simulink model "CR_old"  (R2022a)
settings: Solver=FixedStepDiscrete  StartTime=0.0  StopTime=0.04  FixedStep=0.04  RelTol=1e-3
PreLoadFcn:
  | listing = dir;
  | if (contains([listing .name], 'AGR')) && (contains([listing .name], 'MAP'))
  |     addpath('./AGR', './MAP');
  |     addpath( genpath('./MAP') );
  | elseif (contains([listing .name], 'CR.slx'))
  |     addpath('../AGR', '../MAP');
  |     addpath( genpath('../MAP') );
  | else
  | 
  | end
  | 
  | load('BusStructureCR.mat');
InitFcn:
  | listing = dir;
  | if (contains([listing .name], 'AGR')) && (contains([listing .name], 'MAP'))
  |     addpath('./AGR', './MAP');
  |     addpath( genpath('./MAP') );
  | elseif (contains([listing .name], 'CR.slx'))
  |     addpath('../AGR', '../MAP');
  |     addpath( genpath('../MAP') );
  | else
  | 
  | end
  | 
  | load('BusStructureCR.mat');
StartFcn:
  | listing = dir;
  | if (contains([listing .name], 'AGR')) && (contains([listing .name], 'MAP'))
  |     addpath('./AGR', './MAP');
  |     addpath( genpath('./MAP') );
  | elseif (contains([listing .name], 'CR.slx'))
  |     addpath('../AGR', '../MAP');
  |     addpath( genpath('../MAP') );
  | else
  | 
  | end
  | 
  | load('BusStructureCR.mat');
undefined symbols (not defined in the file): CRDataTag, CRDataTagWrap, CRElevationValid, CRSelected, CRSelectedWraparound, CRTargetElevation, CRTargetLatitude, CRTargetLongitude, CRTargetLOSAvailable, CRTargetLOSAvailableValid, CRValid, deltaECEF, losECEF, nSearch, targetECEF, testLLH
settings Model: Creator=ASCL  LastModifiedBy=ASCL
settings SolverCC: AlgebraicLoopSolver=TrustRegion
settings DataIOCC: SaveOutput=off  SignalLogging=off  DSMLogging=off  SaveTime=off  ReturnWorkspaceOutputs=off
settings OptimizationCC: DefaultParameterBehavior=Inlined  UseDivisionForNetSlopeComputation=on  GainParamInheritBuiltInType=on  UseFloatMulNetSlope=on  InlineInvariantSignals=on  BufferReuse=off  ExpressionFolding=off  PassReuseOutputArgsAs=Individual arguments  ZeroExternalMemoryAtStartup=off  ZeroInternalMemoryAtStartup=off  NoFixptDivByZeroProtection=on  EfficientMapNaN2IntZero=off  LifeSpan=1  EfficientTunableParamExpr=on
settings DebuggingCC: ParameterTunabilityLossMsg=error  UnconnectedInputMsg=warning  UnconnectedOutputMsg=warning  UnconnectedLineMsg=warning  SFMachineParentedDataDiag=warning  ArithmeticOperatorsInVariantConditions=warning
settings HardwareCC: ProdBitPerPointer=32  ProdBitPerSizeT=32  ProdBitPerPtrDiffT=32  ProdLargestAtomicInteger=Long  ProdLargestAtomicFloat=Double  ProdEndianess=BigEndian  ProdWordSize=32  ProdLongLongMode=on  ProdHWDeviceType=Freescale->MPC83xx
settings ModelReferenceCC: ModelReferenceNumInstancesAllowed=Single
settings SFSimCC: SimUserLibraries=MAPd.lib WS2_32.lib  SimUseLocalCustomCode=off  MATLABDynamicMemAlloc=off  CustomCodeUndefinedFunction=UseInterfaceOnly
settings SFSimCC: SimCustomHeaderCode=|
  | #include "MAP.h"
  | #include "MAPDATA.h"
  | #include "DVOF.h"
  | #include "userDefined.h"
settings SFSimCC: SimUserSources=|
  | MAP.c
  | DVOF.c
  | userDefined.c
settings RTWCC: SystemTargetFile=ert.tlc  TemplateMakefile=ert_default_tmf  GenerateReport=on  RTWUseLocalCustomCode=off  RTWUseSimCustomCode=on  CustomLibrary=MAPd.lib WS2_32.lib  IncludeHyperlinkInReport=on  LaunchReport=on  GenerateTraceInfo=on  GenerateTraceReport=on  GenerateTraceReportSl=on  GenerateTraceReportSf=on  GenerateTraceReportEml=on  GenerateCodeMetricsReport=on
settings RTWCC: CustomHeaderCode=|
  | #include "MAP.h"
  | #include "MAPDATA.h"
  | #include "DVOF.h"
  | #include "userDefined.h"
settings RTWCC: CustomSource=|
  | MAP.c
  | DVOF.c
  | userDefined.c
settings CodeAppCC: ForceParamTrailComments=on  IgnoreCustomStorageClasses=off  OperatorAnnotations=on  SimulinkDataObjDesc=on  SFDataObjDesc=on  InsertBlockDesc=on
settings ERTTargetCC: TargetLangStandard=C99 (ISO)  UtilityFuncGeneration=Shared location  GenerateSampleERTMain=on  IncludeMdlTerminateFcn=off  CombineSignalStateStructs=on  SuppressErrorStatus=on  SupportAbsoluteTime=off  SupportComplex=off  InlinedParameterPlacement=NonHierarchical  ERTCustomFileTemplate=example_file_process.tlc  ERTFilePackagingFormat=CompactWithDataFile  EnableSignedLeftShifts=off  EnableSignedRightShifts=off

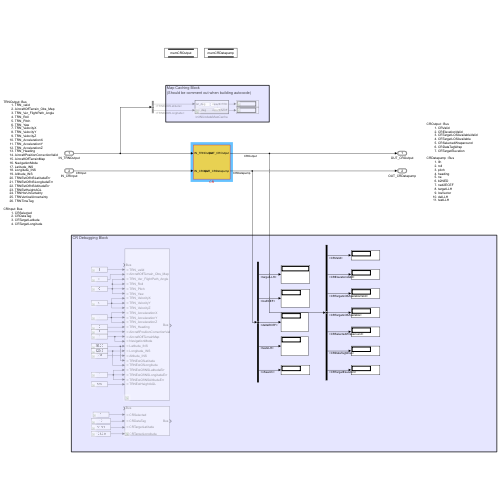
[thumbnail: Simulink's stored preview of the top-level diagram]
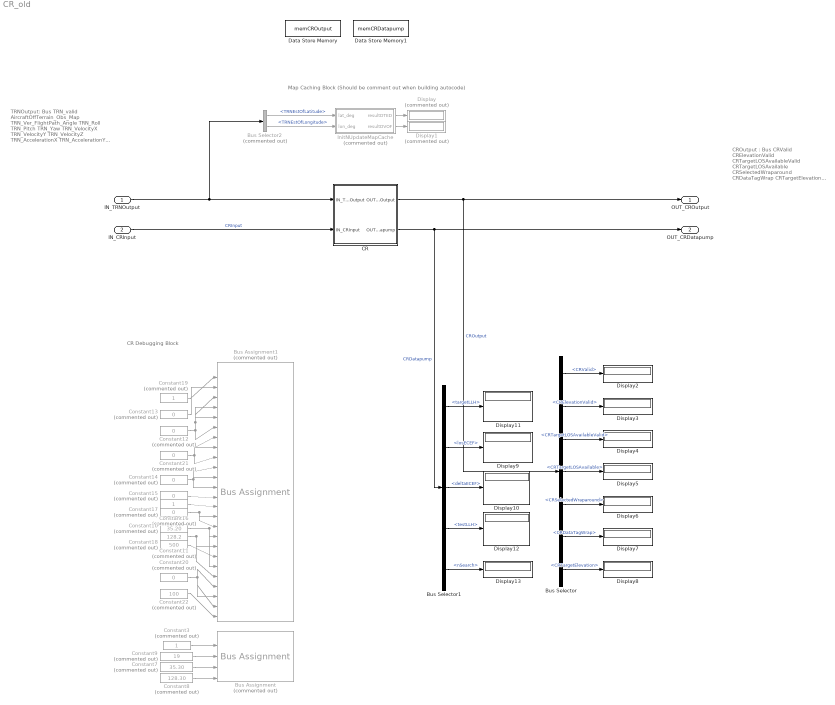
== system CR_old ==
  note: Map Caching Block
      | (Should be comment out when building autocode)
  note: TRNOutput: Bus
      | TRN_valid
      | AircraftOffTerrain_Obs_Map
      | TRN_Ver_FlightPath_Angle
      | TRN_Roll
      | TRN_Pitch
      | TRN_Yaw
      | TRN_VelocityX
      | TRN_VelocityY
      | TRN_VelocityZ
      | TRN_AccelerationX
      | TRN_AccelerationY
      | TRN_AccelerationZ
      | TRN_Heading
      | AircraftPositionCorrectionValid
      | AircraftOffTerrainMap
      | NavigationMode
      | Latitude_INS
      | Longitude_INS
      | Altitude_INS
      | TRNEstOfINSLatitudeErr
      | TRNEstOfINSLongitudeErr
      | TRNEstOfINSAltitudeErr
      | TRNEstHeightAGL
      | TRNHorUncertainty
      | TRNVerticalUncertainty
      | TRNTimeTag
      |
      | CRInput: Bus
      | CRSelected
      | CRDataTag
      | CRTargetLatitude
      | CRTargetLongitude
  note: CROutput : Bus
      | CRValid
      | CRElevationValid
      | CRTargetLOSAvailableValid
      | CRTargetLOSAvailable
      | CRSelectedWraparound
      | CRDataTagWrap
      | CRTargetElevation
      |
      | CRDatapump : Bus
      | llh
      | roll
      | pitch
      | heading
      | ne
      | b2NED
      | ned2ECEF
      | targetLLH
      | losVector
      | delLLH
      | testLLH
  note: CR Debugging Block
  IN_TRNOutput : Inport  OutDataTypeStr=Bus: TRNOutput  BusOutputAsStruct=on
  IN_CRInput : Inport  Port=2  OutDataTypeStr=Bus: CRInput  BusOutputAsStruct=on
  Bus Assignment : BusAssignment  Commented=on  AssignedSignals=CRSelected,CRDataTag,CRTargetLatitude,CRTargetLongitude
  Bus Assignment1 : BusAssignment  Commented=on  AssignedSignals=TRN_valid,AircraftOffTerrain_Obs_Map,TRN_Ver_FlightPath_Angle,TRN_Roll,TRN_Pitch,TRN_Yaw,TRN_VelocityX,TRN_VelocityY,TRN_VelocityZ,TRN_AccelerationX,TRN_AccelerationY,TRN_AccelerationZ,TRN_Heading,AircraftPositionCorrectionValid,AircraftOffTerrainMap,NavigationMode,Latitude_INS,Longitude_INS,Altitude_INS,TRNEstOfLatitude,TRNEstOfLongitude,TRNEstOfINSLatitudeErr,TRNEstOfINSLongitudeErr,TRNEstOfINSAltitudeErr,TRNEstHeightAGL
  Bus Selector : BusSelector  OutputSignals=CRValid,CRElevationValid,CRTargetLOSAvailableValid,CRTargetLOSAvailable,CRSelectedWraparound,CRDataTagWrap,CRTargetElevation
  Bus Selector1 : BusSelector  OutputSignals=targetLLH,losECEF,deltaECEF,testLLH,nSearch
  Bus Selector2 : BusSelector  Commented=on  OutputSignals=TRNEstOfLatitude,TRNEstOfLongitude
  CR : Subsystem
      mask init:
      | % latGPS = double(0);
      | % lonGPS = double(0);
      | % altGPS = double(0);
      | % velEGPS = double(0);
      | % velNGPS = double(0);
      | % velUGPS = double(0);
      | % notValidGPS = boolean(0);
      | % notAvaildINS = boolean(0);
      | % velUINS = double(0);
      | % velVINS = double(0);
      | % velWINS = double(0);
      | % rollINS = double(0);
      | % pitchINS = double(0);
      | % hgdINS = double(0);
      | % accXINS = double(0);
      | % accYINS = double(0);
      | % accZINS = double(0);
      | % activated = boolean(0);
      | % reactionT = uint16(0);
      | % pullUpG = uint16(0);
      | % rollRate = uint16(0);
      | % gOnsetRate = uint16(0);
      | % maxGamma = uint16(0);
      | % setWarnH = double(0);
      | % obsWarningTime = uint16(1);
      | % wiresWarningTime = uint16(1);
      | % latErrOfINS = double(0);
      | % lonErrOfINS = double(0);
      | % altErrorofINS = uint16(0);
      | % heightEstOfTRN = uint16(0);
      | % horUncertaintyOfTRN = double(0);
      | % verUncertaintyOfTRN = double(0);
  Constant10 : Constant  Commented=on  Value=35.20
  Constant11 : Constant  Commented=on  Value=128.2
  Constant{12,14..15,20..21} (5 alike) : Constant  Commented=on  Value=0
  Constant13 : Constant  Commented=on  Value=0  OutDataTypeStr=boolean
  Constant16 : Constant  Commented=on  OutDataTypeStr=boolean
  Constant17 : Constant  Commented=on  Value=0  OutDataTypeStr=boolean
  Constant18 : Constant  Commented=on  Value=500
  Constant19 : Constant  Commented=on  OutDataTypeStr=boolean
  Constant22 : Constant  Commented=on  Value=100  OutDataTypeStr=uint16
  Constant3 : Constant  Commented=on  OutDataTypeStr=boolean
  Constant7 : Constant  Commented=on  Value=35.30
  Constant8 : Constant  Commented=on  Value=128.30
  Constant9 : Constant  Commented=on  Value=19  OutDataTypeStr=uint16
  Data Store Memory : DataStoreMemory  DataStoreName=memCROutput  WriteAfterWriteMsg=warning  ShowAdditionalParam=off  OutDataTypeStr=Bus: CROutput
  Data Store Memory1 : DataStoreMemory  DataStoreName=memCRDatapump  WriteAfterWriteMsg=warning  ShowAdditionalParam=off  OutDataTypeStr=Bus: CRDatapump
  Display : Display  Commented=on
  Display1 : Display  Commented=on
  Display{2..13} (12 alike) : Display
  InitNUpdateMapCache : Subsystem  Commented=on  TreatAsAtomicUnit=on
  OUT_CROutput : Outport  OutDataTypeStr=Bus: CROutput  VectorParamsAs1DForOutWhenUnconnected=off  BusOutputAsStruct=on
  OUT_CRDatapump : Outport  Port=2  OutDataTypeStr=Bus: CRDatapump  VectorParamsAs1DForOutWhenUnconnected=off  BusOutputAsStruct=on
  wires:
  CR/2(OUT_CRDatapump) -> Bus Selector1/1, OUT_CRDatapump/1  "CRDatapump"
  CR/1(OUT_CROutput) -> Bus Selector/1, OUT_CROutput/1  "CROutput"
  InitNUpdateMapCache/1(resultDTED) -> Display/1
  InitNUpdateMapCache/2(resultDVOF) -> Display1/1
  Bus Selector/1 -> Display2/1  "<CRValid>"
  Bus Selector/3 -> Display4/1  "<CRTargetLOSAvailableValid>"
  Bus Selector/2 -> Display3/1  "<CRElevationValid>"
  Bus Selector/7 -> Display8/1  "<CRTargetElevation>"
  Bus Selector/6 -> Display7/1  "<CRDataTagWrap>"
  Bus Selector/5 -> Display6/1  "<CRSelectedWraparound>"
  Bus Selector/4 -> Display5/1  "<CRTargetLOSAvailable>"
  Bus Selector1/2 -> Display9/1  "<losECEF>"
  Bus Selector1/3 -> Display10/1  "<deltaECEF>"
  Bus Selector1/1 -> Display11/1  "<targetLLH>"
  Constant15/1 -> Bus Assignment1/14
  Constant14/1 -> Bus Assignment1/13, Bus Assignment1/11, Bus Assignment1/12
  Constant18/1 -> Bus Assignment1/20
  Constant19/1 -> Bus Assignment1/2
  Constant13/1 -> Bus Assignment1/3
  Constant11/1 -> Bus Assignment1/22, Bus Assignment1/19
  Constant12/1 -> Bus Assignment1/7, Bus Assignment1/4, Bus Assignment1/5, Bus Assignment1/6
  Constant20/1 -> Bus Assignment1/23, Bus Assignment1/25, Bus Assignment1/24
  Constant16/1 -> Bus Assignment1/15
  Constant17/1 -> Bus Assignment1/17, Bus Assignment1/16
  Constant21/1 -> Bus Assignment1/10, Bus Assignment1/8, Bus Assignment1/9
  Constant22/1 -> Bus Assignment1/26
  Constant10/1 -> Bus Assignment1/21, Bus Assignment1/18
  Bus Selector2/1 -> InitNUpdateMapCache/1(lat_deg)  "<TRNEstOfLatitude>"
  Bus Selector2/2 -> InitNUpdateMapCache/2(lon_deg)  "<TRNEstOfLongitude>"
  Constant3/1 -> Bus Assignment/2
  Constant7/1 -> Bus Assignment/4
  Constant8/1 -> Bus Assignment/5
  Constant9/1 -> Bus Assignment/3
  IN_TRNOutput/1 -> Bus Selector2/1, CR/1(IN_TRNOutput)
  IN_CRInput/1 -> CR/2(IN_CRInput)  "CRInput"
  Bus Selector1/4 -> Display12/1  "<testLLH>"
  Bus Selector1/5 -> Display13/1  "<nSearch>"

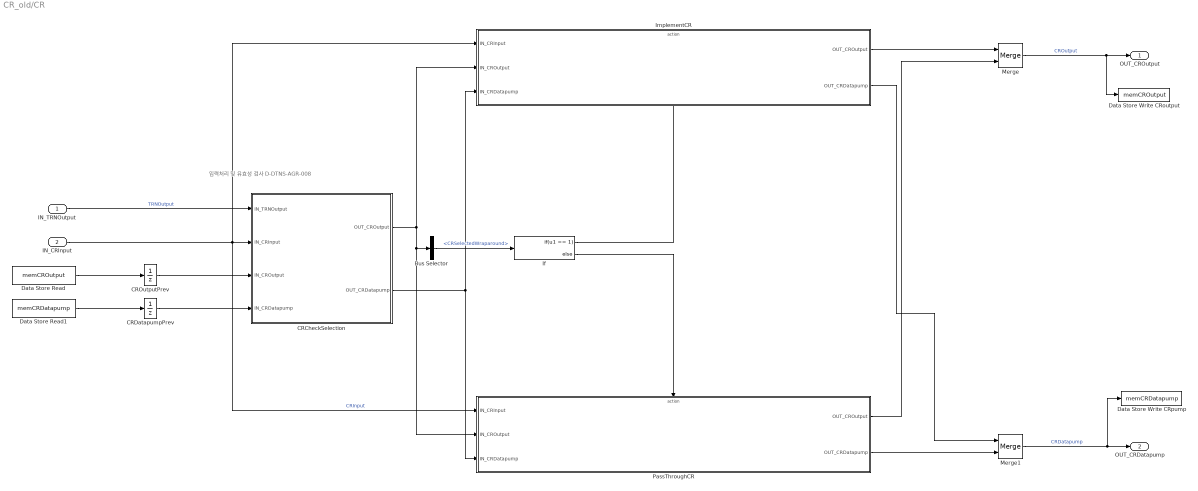
== system CR_old/CR ==
  note: 입력처리 및 유효성 검사 D-DTNS-AGR-008
  IN_TRNOutput : Inport  OutDataTypeStr=Bus: TRNOutput
  IN_CRInput : Inport  Port=2  OutDataTypeStr=Bus: CRInput
  Bus Selector : BusSelector  OutputSignals=CRSelectedWraparound
  CRCheckSelection : Subsystem  TreatAsAtomicUnit=on
      settings: RTWSystemCode=Nonreusable function  RTWFcnNameOpts=Use subsystem name
  CRDatapumpPrev : UnitDelay  SampleTime=-1  HasFrameUpgradeWarning=on
  CROutputPrev : UnitDelay  SampleTime=-1  HasFrameUpgradeWarning=on
  Data Store Read : DataStoreRead  DataStoreName=memCROutput  IndexOptions=Index vector (dialog)  Indices=1  OutputSizes=1
  Data Store Read1 : DataStoreRead  DataStoreName=memCRDatapump  IndexOptions=Index vector (dialog)  Indices=1  OutputSizes=1
  Data Store Write CRoutput : DataStoreWrite  DataStoreName=memCROutput  IndexOptions=Index vector (dialog)  Indices=1  OutputSizes=1
  Data Store Write CRpump : DataStoreWrite  DataStoreName=memCRDatapump  IndexOptions=Index vector (dialog)  Indices=1  OutputSizes=1
  If : If  IfExpression=u1 == 1
  ImplementCR : Subsystem  TreatAsAtomicUnit=on
      settings: RTWSystemCode=Nonreusable function  RTWFcnNameOpts=Use subsystem name
  Merge : Merge
  Merge1 : Merge
  PassThroughCR : Subsystem  TreatAsAtomicUnit=on
      settings: RTWSystemCode=Nonreusable function  RTWFcnNameOpts=Use subsystem name
  OUT_CROutput : Outport  OutDataTypeStr=Bus: CROutput  VectorParamsAs1DForOutWhenUnconnected=off
  OUT_CRDatapump : Outport  Port=2  OutDataTypeStr=Bus: CRDatapump  VectorParamsAs1DForOutWhenUnconnected=off
  wires:
  IN_CRInput/1 -> ImplementCR/1(IN_CRInput), PassThroughCR/1(IN_CRInput), CRCheckSelection/2(IN_CRInput)  "CRInput"
  Merge/1 -> OUT_CROutput/1, Data Store Write CRoutput/1  "CROutput"
  Merge1/1 -> Data Store Write CRpump/1, OUT_CRDatapump/1  "CRDatapump"
  Data Store Read/1 -> CROutputPrev/1
  Data Store Read1/1 -> CRDatapumpPrev/1
  ImplementCR/1(OUT_CROutput) -> Merge/1
  PassThroughCR/2(OUT_CRDatapump) -> Merge1/2
  ImplementCR/2(OUT_CRDatapump) -> Merge1/1
  PassThroughCR/1(OUT_CROutput) -> Merge/2
  CRCheckSelection/1(OUT_CROutput) -> Bus Selector/1, PassThroughCR/2(IN_CROutput), ImplementCR/2(IN_CROutput)
  CRCheckSelection/2(OUT_CRDatapump) -> PassThroughCR/3(IN_CRDatapump), ImplementCR/3(IN_CRDatapump)
  Bus Selector/1 -> If/1  "<CRSelectedWraparound>"
  If/1 -> ImplementCR/Action
  If/2 -> PassThroughCR/Action
  IN_TRNOutput/1 -> CRCheckSelection/1(IN_TRNOutput)  "TRNOutput"
  CROutputPrev/1 -> CRCheckSelection/3(IN_CROutput)
  CRDatapumpPrev/1 -> CRCheckSelection/4(IN_CRDatapump)

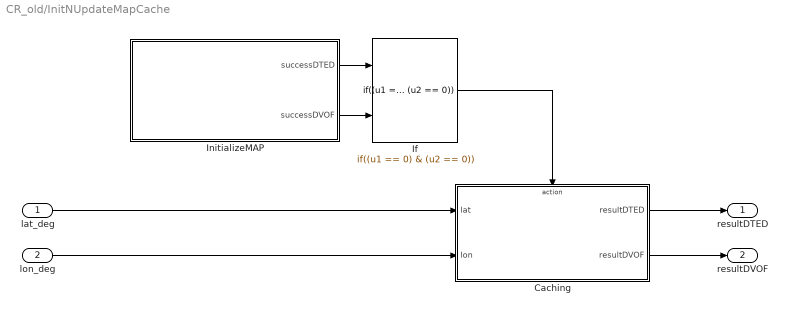
== system CR_old/InitNUpdateMapCache ==
  lat_deg : Inport
  lon_deg : Inport  Port=2
  Caching : Subsystem  TreatAsAtomicUnit=on
  If : If  NumInputs=2  IfExpression=(u1 == 0) & (u2 == 0)  ShowElse=off
  InitializeMAP : MATLAB Function  TreatAsAtomicUnit=on
  resultDTED : Outport  VectorParamsAs1DForOutWhenUnconnected=off
  resultDVOF : Outport  Port=2  VectorParamsAs1DForOutWhenUnconnected=off
  wires:
  Caching/1(resultDTED) -> resultDTED/1
  InitializeMAP/1(successDTED) -> If/1
  Caching/2(resultDVOF) -> resultDVOF/1
  InitializeMAP/2(successDVOF) -> If/2
  If/1 -> Caching/Action
  lat_deg/1 -> Caching/1(lat)
  lon_deg/1 -> Caching/2(lon)

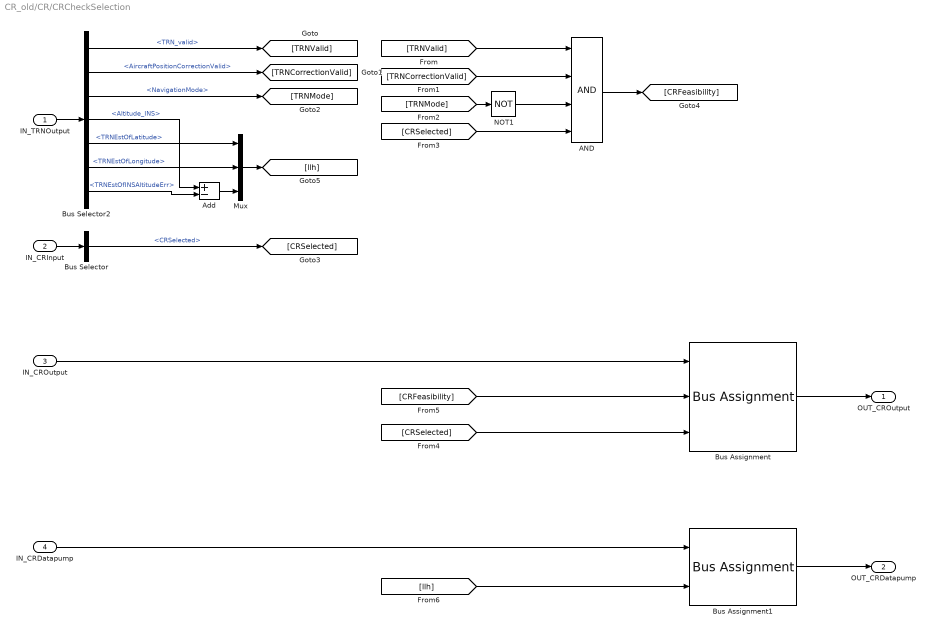
== system CR_old/CR/CRCheckSelection ==
  IN_TRNOutput : Inport  OutDataTypeStr=Bus: TRNOutput
  IN_CRInput : Inport  Port=2  OutDataTypeStr=Bus: CRInput
  IN_CROutput : Inport  Port=3  OutDataTypeStr=Bus: CROutput
  IN_CRDatapump : Inport  Port=4  OutDataTypeStr=Bus: CRDatapump
  AND : Logic  Inputs=4  AllPortsSameDT=off  OutDataTypeStr=boolean
  Add : Sum  Inputs=+-
  Bus Assignment : BusAssignment  AssignedSignals=CRValid,CRSelectedWraparound
  Bus Assignment1 : BusAssignment  AssignedSignals=llh
  Bus Selector : BusSelector  OutputSignals=CRSelected
  Bus Selector2 : BusSelector  OutputSignals=TRN_valid,AircraftPositionCorrectionValid,NavigationMode,Altitude_INS,TRNEstOfLatitude,TRNEstOfLongitude,TRNEstOfINSAltitudeErr
  Mux : Mux  Inputs=3
  NOT1 : Logic  Operator=NOT  IconShape=distinctive  AllPortsSameDT=off  OutDataTypeStr=boolean
  OUT_CROutput : Outport  OutDataTypeStr=Bus: CROutput  VectorParamsAs1DForOutWhenUnconnected=off
  OUT_CRDatapump : Outport  Port=2  OutDataTypeStr=Bus: CRDatapump  VectorParamsAs1DForOutWhenUnconnected=off
  wires:
  IN_CRInput/1 -> Bus Selector/1
  IN_CROutput/1 -> Bus Assignment/1
  Bus Assignment/1 -> OUT_CROutput/1
  IN_CRDatapump/1 -> Bus Assignment1/1
  Bus Selector/1 -> [CRSelected]  "<CRSelected>"
  IN_TRNOutput/1 -> Bus Selector2/1
  Bus Selector2/2 -> [TRNCorrectionValid]  "<AircraftPositionCorrectionValid>"
  Bus Selector2/3 -> [TRNMode]  "<NavigationMode>"
  Bus Selector2/1 -> [TRNValid]  "<TRN_valid>"
  Bus Selector2/6 -> Mux/2  "<TRNEstOfLongitude>"
  Mux/1 -> [llh]
  Add/1 -> Mux/3
  Bus Selector2/5 -> Mux/1  "<TRNEstOfLatitude>"
  Bus Selector2/4 -> Add/1  "<Altitude_INS>"
  Bus Selector2/7 -> Add/2  "<TRNEstOfINSAltitudeErr>"
  [CRSelected] -> AND/4
  NOT1/1 -> AND/3
  [TRNValid] -> AND/1
  [TRNCorrectionValid] -> AND/2
  [TRNMode] -> NOT1/1
  AND/1 -> [CRFeasibility]
  [CRSelected] -> Bus Assignment/3
  [CRFeasibility] -> Bus Assignment/2
  Bus Assignment1/1 -> OUT_CRDatapump/1
  [llh] -> Bus Assignment1/2

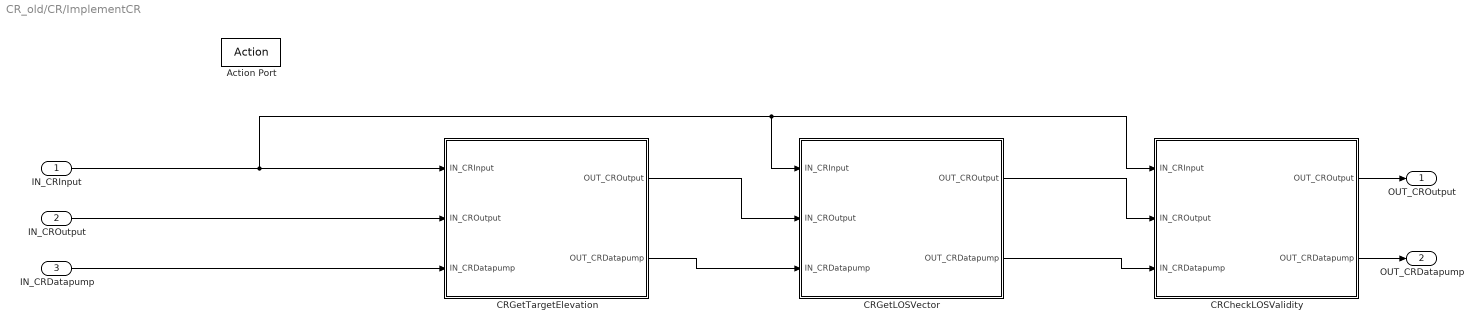
== system CR_old/CR/ImplementCR ==
  IN_CRInput : Inport  OutDataTypeStr=Bus: CRInput
  IN_CROutput : Inport  Port=2  OutDataTypeStr=Bus: CROutput
  IN_CRDatapump : Inport  Port=3  OutDataTypeStr=Bus: CRDatapump
  Action Port : ActionPort  ActionPortLabel=if(u1 == 1)
  CRCheckLOSValidity : Subsystem  TreatAsAtomicUnit=on
      settings: RTWSystemCode=Nonreusable function  RTWFcnNameOpts=Use subsystem name
  CRGetLOSVector : Subsystem  TreatAsAtomicUnit=on
      settings: RTWSystemCode=Nonreusable function  RTWFcnNameOpts=Use subsystem name
  CRGetTargetElevation : Subsystem  TreatAsAtomicUnit=on
      settings: RTWSystemCode=Nonreusable function  RTWFcnNameOpts=Use subsystem name
  OUT_CROutput : Outport  OutDataTypeStr=Bus: CROutput  VectorParamsAs1DForOutWhenUnconnected=off
  OUT_CRDatapump : Outport  Port=2  OutDataTypeStr=Bus: CRDatapump  VectorParamsAs1DForOutWhenUnconnected=off
  wires:
  CRGetLOSVector/2(OUT_CRDatapump) -> CRCheckLOSValidity/3(IN_CRDatapump)
  IN_CRDatapump/1 -> CRGetTargetElevation/3(IN_CRDatapump)
  CRGetTargetElevation/2(OUT_CRDatapump) -> CRGetLOSVector/3(IN_CRDatapump)
  IN_CRInput/1 -> CRCheckLOSValidity/1(IN_CRInput), CRGetLOSVector/1(IN_CRInput), CRGetTargetElevation/1(IN_CRInput)
  IN_CROutput/1 -> CRGetTargetElevation/2(IN_CROutput)
  CRGetTargetElevation/1(OUT_CROutput) -> CRGetLOSVector/2(IN_CROutput)
  CRGetLOSVector/1(OUT_CROutput) -> CRCheckLOSValidity/2(IN_CROutput)
  CRCheckLOSValidity/1(OUT_CROutput) -> OUT_CROutput/1
  CRCheckLOSValidity/2(OUT_CRDatapump) -> OUT_CRDatapump/1

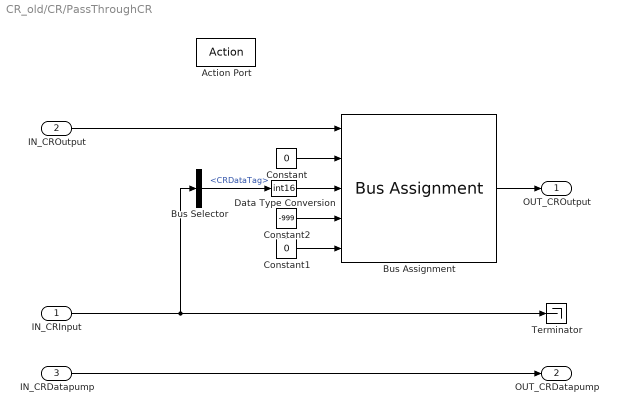
== system CR_old/CR/PassThroughCR ==
  IN_CRInput : Inport  OutDataTypeStr=Bus: CRInput
  IN_CROutput : Inport  Port=2  OutDataTypeStr=Bus: CROutput
  IN_CRDatapump : Inport  Port=3  OutDataTypeStr=Bus: CRDatapump
  Action Port : ActionPort  ActionPortLabel=else
  Bus Assignment : BusAssignment  AssignedSignals=CRValid,CRDataTagWrap,CRTargetElevation,CRElevationValid
  Bus Selector : BusSelector  OutputSignals=CRDataTag
  Constant : Constant  Value=0  OutDataTypeStr=boolean
  Constant1 : Constant  Value=0  OutDataTypeStr=boolean
  Constant2 : Constant  Value=-999  OutDataTypeStr=int16
  Data Type Conversion : DataTypeConversion  OutDataTypeStr=int16  SaturateOnIntegerOverflow=off  RndMeth=Floor
  Terminator : Terminator
  OUT_CROutput : Outport  OutDataTypeStr=Bus: CROutput  VectorParamsAs1DForOutWhenUnconnected=off
  OUT_CRDatapump : Outport  Port=2  OutDataTypeStr=Bus: CRDatapump  VectorParamsAs1DForOutWhenUnconnected=off
  wires:
  IN_CROutput/1 -> Bus Assignment/1
  IN_CRDatapump/1 -> OUT_CRDatapump/1
  IN_CRInput/1 -> Bus Selector/1, Terminator/1
  Constant/1 -> Bus Assignment/2
  Bus Assignment/1 -> OUT_CROutput/1
  Bus Selector/1 -> Data Type Conversion/1  "<CRDataTag>"
  Data Type Conversion/1 -> Bus Assignment/3
  Constant1/1 -> Bus Assignment/5
  Constant2/1 -> Bus Assignment/4

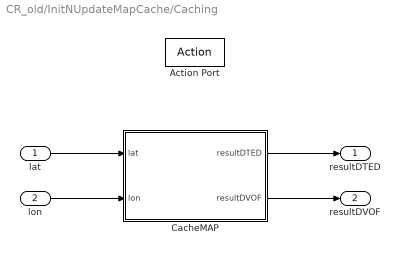
== system CR_old/InitNUpdateMapCache/Caching ==
  lat : Inport
  lon : Inport  Port=2
  Action Port : ActionPort  ActionPortLabel=if((u1 == 0) & (u2 == 0))
  CacheMAP : MATLAB Function  TreatAsAtomicUnit=on
  resultDTED : Outport  VectorParamsAs1DForOutWhenUnconnected=off
  resultDVOF : Outport  Port=2  VectorParamsAs1DForOutWhenUnconnected=off
  wires:
  CacheMAP/1(resultDTED) -> resultDTED/1
  lat/1 -> CacheMAP/1(lat)
  lon/1 -> CacheMAP/2(lon)
  CacheMAP/2(resultDVOF) -> resultDVOF/1

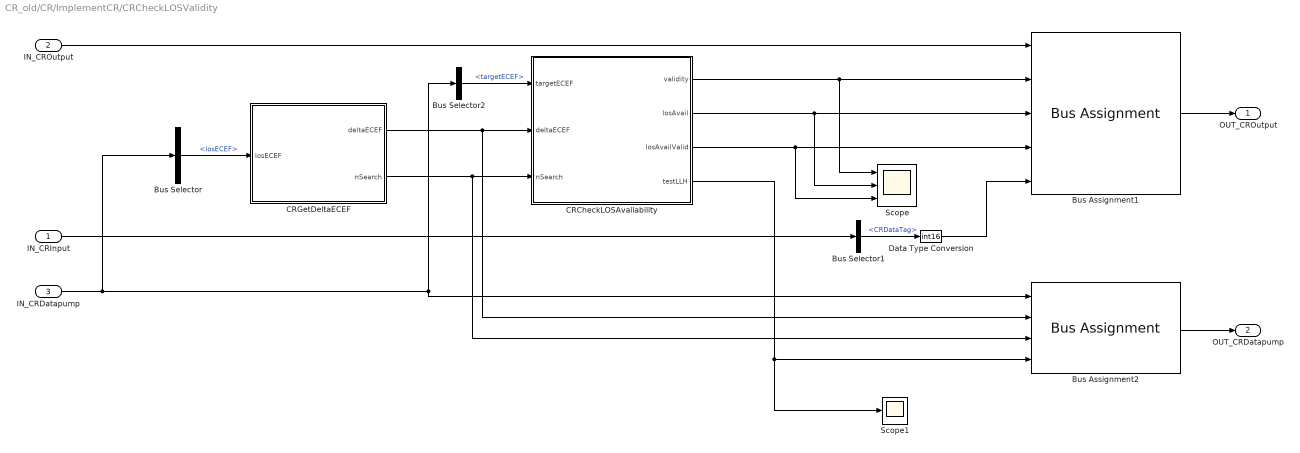
== system CR_old/CR/ImplementCR/CRCheckLOSValidity ==
  IN_CRInput : Inport  OutDataTypeStr=Bus: CRInput
  IN_CROutput : Inport  Port=2  OutDataTypeStr=Bus: CROutput
  IN_CRDatapump : Inport  Port=3  OutDataTypeStr=Bus: CRDatapump
  Bus Assignment1 : BusAssignment  AssignedSignals=CRValid,CRTargetLOSAvailable,CRTargetLOSAvailableValid,CRDataTagWrap
  Bus Assignment2 : BusAssignment  AssignedSignals=deltaECEF,nSearch,testLLH
  Bus Selector : BusSelector  OutputSignals=losECEF
  Bus Selector1 : BusSelector  OutputSignals=CRDataTag
  Bus Selector2 : BusSelector  OutputSignals=targetECEF
  CRCheckLOSAvailability : MATLAB Function  TreatAsAtomicUnit=on
  CRGetDeltaECEF : MATLAB Function  TreatAsAtomicUnit=on
  Data Type Conversion : DataTypeConversion  OutDataTypeStr=int16  SaturateOnIntegerOverflow=off  RndMeth=Floor
  Scope : Scope  NumInputPorts=3
  Scope1 : Scope
  OUT_CROutput : Outport  OutDataTypeStr=Bus: CROutput  VectorParamsAs1DForOutWhenUnconnected=off
  OUT_CRDatapump : Outport  Port=2  OutDataTypeStr=Bus: CRDatapump  VectorParamsAs1DForOutWhenUnconnected=off
  wires:
  IN_CRInput/1 -> Bus Selector1/1
  IN_CROutput/1 -> Bus Assignment1/1
  Bus Assignment1/1 -> OUT_CROutput/1
  IN_CRDatapump/1 -> Bus Selector2/1, Bus Assignment2/1, Bus Selector/1
  Bus Selector1/1 -> Data Type Conversion/1  "<CRDataTag>"
  Data Type Conversion/1 -> Bus Assignment1/5
  CRCheckLOSAvailability/1(validity) -> Scope/1, Bus Assignment1/2
  CRCheckLOSAvailability/2(losAvail) -> Bus Assignment1/3, Scope/2
  CRCheckLOSAvailability/3(losAvailValid) -> Scope/3, Bus Assignment1/4
  Bus Assignment2/1 -> OUT_CRDatapump/1
  CRCheckLOSAvailability/4(testLLH) -> Bus Assignment2/4, Scope1/1
  Bus Selector/1 -> CRGetDeltaECEF/1(losECEF)  "<losECEF>"
  CRGetDeltaECEF/1(deltaECEF) -> CRCheckLOSAvailability/2(deltaECEF), Bus Assignment2/2
  CRGetDeltaECEF/2(nSearch) -> CRCheckLOSAvailability/3(nSearch), Bus Assignment2/3
  Bus Selector2/1 -> CRCheckLOSAvailability/1(targetECEF)  "<targetECEF>"

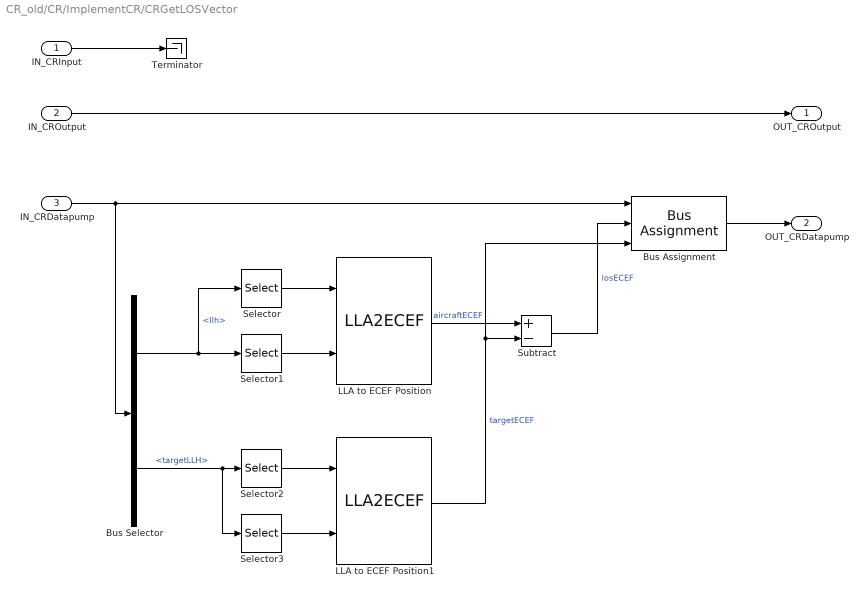
== system CR_old/CR/ImplementCR/CRGetLOSVector ==
  IN_CRInput : Inport  OutDataTypeStr=Bus: CRInput
  IN_CROutput : Inport  Port=2  OutDataTypeStr=Bus: CROutput
  IN_CRDatapump : Inport  Port=3  OutDataTypeStr=Bus: CRDatapump
  Bus Assignment : BusAssignment  AssignedSignals=losECEF,targetECEF
  Bus Selector : BusSelector  OutputSignals=llh,targetLLH
  LLA to ECEF Position : LLA2ECEF
  LLA to ECEF Position1 : LLA2ECEF
  Selector : Selector  IndexMode=Zero-based  InputPortWidth=3  IndexOptions=Index vector (dialog)  Indices=[0 1]  OutputSizes=1
  Selector1 : Selector  IndexMode=Zero-based  InputPortWidth=3  IndexOptions=Index vector (dialog)  Indices=[2]  OutputSizes=1
  Selector2 : Selector  IndexMode=Zero-based  InputPortWidth=3  IndexOptions=Index vector (dialog)  Indices=[0 1]  OutputSizes=1
  Selector3 : Selector  IndexMode=Zero-based  InputPortWidth=3  IndexOptions=Index vector (dialog)  Indices=[2]  OutputSizes=1
  Subtract : Sum  Inputs=+-
  Terminator : Terminator
  OUT_CROutput : Outport  OutDataTypeStr=Bus: CROutput  VectorParamsAs1DForOutWhenUnconnected=off
  OUT_CRDatapump : Outport  Port=2  OutDataTypeStr=Bus: CRDatapump  VectorParamsAs1DForOutWhenUnconnected=off
  wires:
  IN_CRDatapump/1 -> Bus Selector/1, Bus Assignment/1
  IN_CRInput/1 -> Terminator/1
  Bus Assignment/1 -> OUT_CRDatapump/1
  IN_CROutput/1 -> OUT_CROutput/1
  Bus Selector/1 -> Selector/1, Selector1/1  "<llh>"
  Bus Selector/2 -> Selector3/1, Selector2/1  "<targetLLH>"
  Subtract/1 -> Bus Assignment/2  "losECEF"
  Selector/1 -> LLA to ECEF Position/1
  Selector1/1 -> LLA to ECEF Position/2
  Selector2/1 -> LLA to ECEF Position1/1
  Selector3/1 -> LLA to ECEF Position1/2
  LLA to ECEF Position/1 -> Subtract/1  "aircraftECEF"
  LLA to ECEF Position1/1 -> Bus Assignment/3, Subtract/2  "targetECEF"

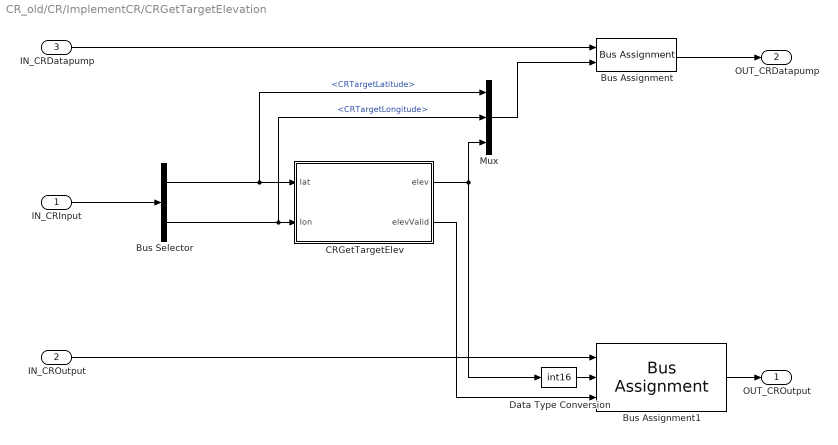
== system CR_old/CR/ImplementCR/CRGetTargetElevation ==
  IN_CRInput : Inport  OutDataTypeStr=Bus: CRInput
  IN_CROutput : Inport  Port=2  OutDataTypeStr=Bus: CROutput
  IN_CRDatapump : Inport  Port=3  OutDataTypeStr=Bus: CRDatapump
  Bus Assignment : BusAssignment  AssignedSignals=targetLLH
  Bus Assignment1 : BusAssignment  AssignedSignals=CRTargetElevation,CRElevationValid
  Bus Selector : BusSelector  OutputSignals=CRTargetLatitude,CRTargetLongitude
  CRGetTargetElev : MATLAB Function  TreatAsAtomicUnit=on
  Data Type Conversion : DataTypeConversion  OutDataTypeStr=int16  SaturateOnIntegerOverflow=off  RndMeth=Floor
  Mux : Mux  Inputs=3
  OUT_CROutput : Outport  OutDataTypeStr=Bus: CROutput  VectorParamsAs1DForOutWhenUnconnected=off
  OUT_CRDatapump : Outport  Port=2  OutDataTypeStr=Bus: CRDatapump  VectorParamsAs1DForOutWhenUnconnected=off
  wires:
  IN_CRDatapump/1 -> Bus Assignment/1
  IN_CRInput/1 -> Bus Selector/1
  Bus Selector/1 -> Mux/1, CRGetTargetElev/1(lat)  "<CRTargetLatitude>"
  Bus Selector/2 -> Mux/2, CRGetTargetElev/2(lon)  "<CRTargetLongitude>"
  CRGetTargetElev/1(elev) -> Data Type Conversion/1, Mux/3
  Mux/1 -> Bus Assignment/2
  Bus Assignment/1 -> OUT_CRDatapump/1
  IN_CROutput/1 -> Bus Assignment1/1
  Bus Assignment1/1 -> OUT_CROutput/1
  Data Type Conversion/1 -> Bus Assignment1/2
  CRGetTargetElev/2(elevValid) -> Bus Assignment1/3

== matlab function CR_old/CR/ImplementCR/CRGetTargetElevation/CRGetTargetElev ==
  data: lat input; elev output; lon input; elevValid output
function [elev, elevValid] = CRGetTargetElev(lat, lon)

elev = 0.0;
elevValid = false;

isScanBoundaryFlag = int8(0);
isScanBoundaryFlag = coder.ceval('IsScanBoundary', lat, lon);

if (isScanBoundaryFlag == 1)
    elev = coder.ceval('GetElevation', lat, lon);
    elevValid = true;
else
    elev = -999;
    elevValid = false;
end

== matlab function CR_old/CR/ImplementCR/CRCheckLOSValidity/CRGetDeltaECEF ==
  data: losECEF input; deltaECEF output; nSearch output
function [deltaECEF, nSearch] = CRGetDeltaECEF(losECEF)
%CRGETDELTAECEF
% 
% == Inputs =========
% losECEF           - LOS vector in {ECEF} [m]
% 
% == Outputs ========
% deltaECEF         - Incremental of LOS search vector in {ECEF} [m]
% nSearch           - number of intersection search required
% 

% Define
MIN_DIST = 30.0;

% Initialize
deltaECEF = zeros(3, 1);
nSearch = 2;

% Calculate the distance between A/C and target using los_ECEF vector
tarDistance = norm(losECEF);

% Calculate number of intersection search required
if (tarDistance < MIN_DIST)
    nSearch = 2;
else
    nSearch = ceil(tarDistance/MIN_DIST) + 1;
end

% Calculate the incremental of LOS search vector
deltaECEF = losECEF / (nSearch-1);

end

== matlab function CR_old/CR/ImplementCR/CRCheckLOSValidity/CRCheckLOSAvailability ==
  data: targetECEF input; validity output; losAvail output; losAvailValid output; deltaECEF input; nSearch input; testLLH output
function [validity, losAvail, losAvailValid, testLLH] = CRCheckLOSAvailability(targetECEF, deltaECEF, nSearch)

% Initialization
validity        = false;
losAvail        = false;
losAvailValid   = false;
isMapCached_int = int32(0);
testLLH         = zeros(3, 1);
testTerElev     = 0.0;
testObsElev     = 0.0;
testElev        = 0.0;
index           = 0;
latOut          = 0.0;
lonOut          = 0.0;
AMSLI           = 0;
AMSL            = 0;

for ii=0:(nSearch-1)
    testTerElev = 0.0;
    testObsElev = 0.0;

    % 1. Propagate search vector
    testECEF = targetECEF + (ii * deltaECEF); 
    
    % 2. Convert test ECEF coordinate to LLH
    testLLH = ecef2llh(testECEF);
    
    % 3-1. Check Map data is cached
    isMapCached_int = coder.ceval('IsScanBoundary', testLLH(1), testLLH(2));
    if ( isMapCached_int == 0 )
        losAvailValid = false;
        return
    end
    
    % 3-2. Get Terrain Elevation
    testTerElev = coder.ceval('GetElevation', testLLH(1), testLLH(2));
    
    % 3-3. Get Obstacle Info
    index = coder.ceval('GetObstTotalCount');
    AMSL  = 0;
    if (index >= 0)
        for jj=0:index-1
            latOut = coder.ceval('GetObstacleInfo', testLLH(1), testLLH(2), jj, 1);
            lonOut = coder.ceval('GetObstacleInfo', testLLH(1), testLLH(2), jj, 2);
            dist=sqrt(((testLLH(1)-latOut)*pi/180*6378137)^2+((testLLH(2)-lonOut)*pi/180*6378137)^2);
            if (dist<50)
                AMSLI = coder.ceval('GetObstacleInfo', testLLH(1), testLLH(2), jj, 4);
                if (AMSLI>AMSL)
                    AMSL=AMSLI;
                end
            end
        end
    end
    testObsElev   = AMSL;
    
    % 2-3. Get Highest Profile
    if ( testTerElev > testObsElev )
        testElev = testTerElev;
    else
        testElev = testObsElev;
    end
    
    % 3. Test LOS Availability
    if (testElev > testLLH(3))
        losAvail = false;
        fprintf("LOS NOT AVAILABLE. testElev: %f, testLLH(3): %f \r\n", testElev, testLLH(3));
        return
    else
        
    end

end

validity = true;
losAvail = true;
losAvailValid = true;

end

function llh = ecef2llh(xyzECEF)
%ECEF2LLH
% Compute the {LLH} coordinates given {ECEF}
%
% == Inputs =========
% ecef              - {ECEF} coordinates [m, m, m]
%
% == Outputs ========
% llh               - Corresponding Latitude, Longitude, Height [deg,deg,m]
%

% Initialization
llh = zeros(3,1);

% WGS84 Parameters
r_e     = 6378137.0;
f       = 1/298.257223563;
r_b     = r_e * (1-f);
e       = 0.08181919;

% For convenience
x       = xyzECEF(1); 
y       = xyzECEF(2); 
z       = xyzECEF(3);

% Longitude
lon = atan2(y, x);

% Iteration for Latitude and Height
eps     = 1;
tol     = 1e-10;
p       = sqrt(x^2 + y^2);
lat     = atan(z/(p*(1-e^2)));
h       = 0.0;

while (eps > tol)
    N   = r_e^2 / sqrt(r_e^2*cos(lat)^2 + r_b^2*sin(lat)^2);
    h   = p / cos(lat) - N;
    lat0 = lat;
    lat = atan(z / ( p * ( 1 - e^2*N/(N+h) ) ) );
    eps = abs(lat - lat0);
end

% Parse outputs
llh = [lat*(180/pi); lon*(180/pi); h];


end

== matlab function CR_old/InitNUpdateMapCache/InitializeMAP ==
  data: successDTED output; successDVOF output
function [successDTED, successDVOF] = InitializeMAP()

flagDTED = int32(1);
flagDVOF = int32(1);

pathDTED = 'C:\Users\ASCL\Documents\GitHub\DTNS\MAP\MAP_DB\';
pathDVOF = 'C:\Users\ASCL\Documents\GitHub\DTNS\MAP\DVOF\';

strLenDTED = int32(strlength(pathDTED));
strLenDVOF = int32(strlength(pathDVOF));

flagDTED = coder.ceval('InitialMap', pathDTED, strLenDTED );
flagDVOF = coder.ceval('InitDVOF', pathDVOF, strLenDVOF );

successDTED = flagDTED;
successDVOF = flagDVOF;

== matlab function CR_old/InitNUpdateMapCache/Caching/CacheMAP ==
  data: resultDTED output; resultDVOF output; lat input; lon input
function [resultDTED, resultDVOF] = CacheMAP(lat, lon)

resultDTED = int32(1);
resultDVOF = int32(1);

resultDVOF = coder.ceval('UpdateObstList', lat, lon);
resultDTED = coder.ceval('UpdateMapCache', lat, lon);
